simulink model "proj_30_10"  (R2020a)
settings: Solver=VariableStepAuto  StartTime=0.0  StopTime=10.0  RelTol=1e-3
undefined symbols (not defined in the file): T
settings Model: Creator=jguil  LastModifiedBy=jguil

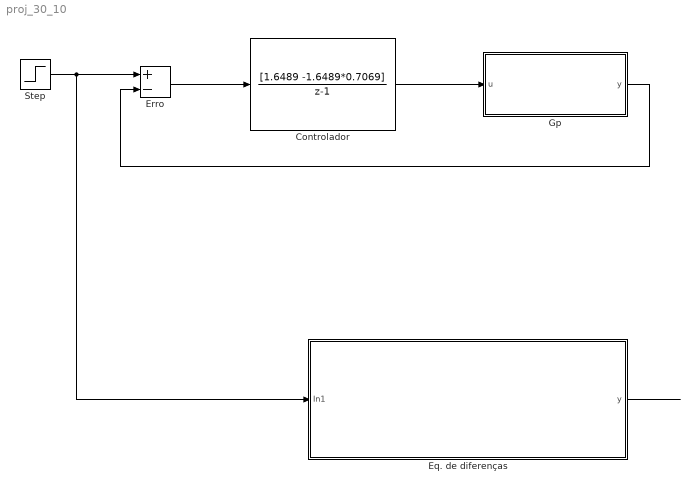
== system proj_30_10 ==
  Controlador : DiscreteTransferFcn  Numerator=[1.6489 -1.6489*0.7069]  Denominator=[1 -1]  SampleTime=T
  Eq. de diferenças : Subsystem
  Erro : Sum  Inputs=+-
  Gp : Subsystem
  Step : Step  SampleTime=0
  wires:
  Erro/1 -> Controlador/1
  Controlador/1 -> Gp/1(u)
  Gp/1(y) -> Erro/2
  Step/1 -> Eq. de diferenças/1(In1), Erro/1
  Eq. de diferenças/1(y) -> ?

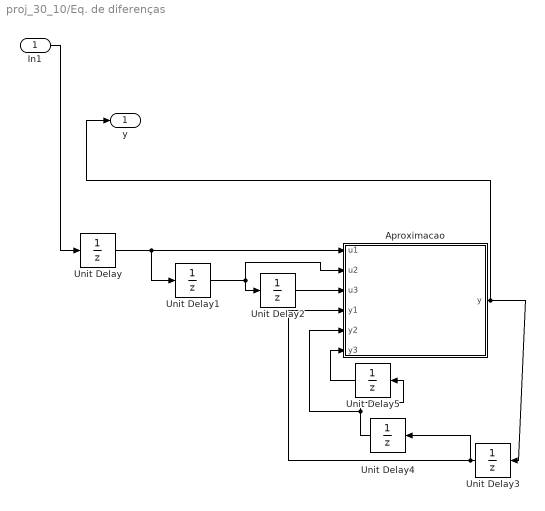
== system proj_30_10/Eq. de diferenças ==
  In1 : Inport
  Aproximacao : MATLAB Function  TreatAsAtomicUnit=on
  Unit Delay{,1..5} (6 alike) : UnitDelay  SampleTime=T  HasFrameUpgradeWarning=on
  y : Outport
  wires:
  Unit Delay2/1 -> Aproximacao/3(u3)
  In1/1 -> Unit Delay/1
  Unit Delay5/1 -> Aproximacao/6(y3)
  Unit Delay3/1 -> Aproximacao/4(y1), Unit Delay4/1
  Aproximacao/1(y) -> y/1, Unit Delay3/1
  Unit Delay4/1 -> Aproximacao/5(y2), Unit Delay5/1
  Unit Delay1/1 -> Aproximacao/2(u2), Unit Delay2/1
  Unit Delay/1 -> Aproximacao/1(u1), Unit Delay1/1

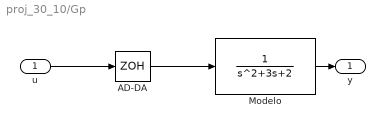
== system proj_30_10/Gp ==
  u : Inport
  AD-DA : ZeroOrderHold  SampleTime=-1
  Modelo : TransferFcn  Denominator=[1 3 2]
  y : Outport
  wires:
  AD-DA/1 -> Modelo/1
  u/1 -> AD-DA/1
  Modelo/1 -> y/1

== matlab function proj_30_10/Eq. de diferenças/Aproximacao ==
  data: u1 input; y output; u2 input; u3 input; y1 input; y2 input; y3 input
function y = aprox(u1,u2,u3,y1,y2,y3)
% y =
% 2.03y(n-1)-1.418y(n-2)+0.3437y(n-3)+0.08961u(n-1)-0.003278u(n-2)-0.04246u(n-3)

y = 2.03*y1 -1.418*y2 +0.3437*y3 +0.08961*u1 -0.003278*u2 -0.04246*u3;
